simulink model "bolide_complet"  (R2023b)
settings: Solver=VariableStepAuto  StartTime=0.0  StopTime=50  RelTol=1e-3
model workspace (MATLAB code in the model file):
  | % Paramètres du système
  | mb = 0.7;
  | mw = 0.1;
  | Ix = 0.001;
  | Iz = 0.001;
  | Iwx = 0.001;
  | Iwy = 0.001;
  | Iwz = 0.001;
  | l = 0.22;
  | d = 0.2;
  | R = 2.05;
  | k = 0.258;
  | rho = 0.04;
  | 
  | % A l'équilibre
  | 
  | ubar = 1;
  | psibar = 0;
libraries: slpidlib x2

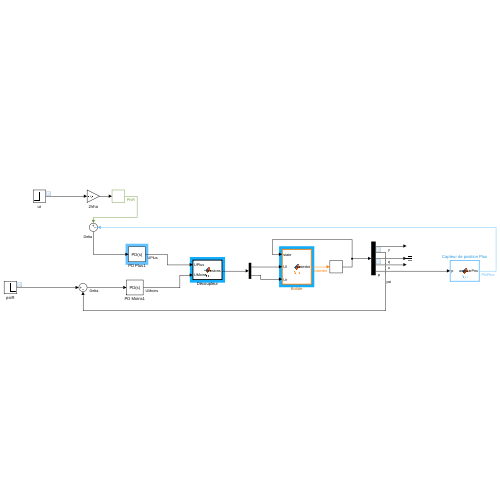
[thumbnail: Simulink's stored preview of the top-level diagram]
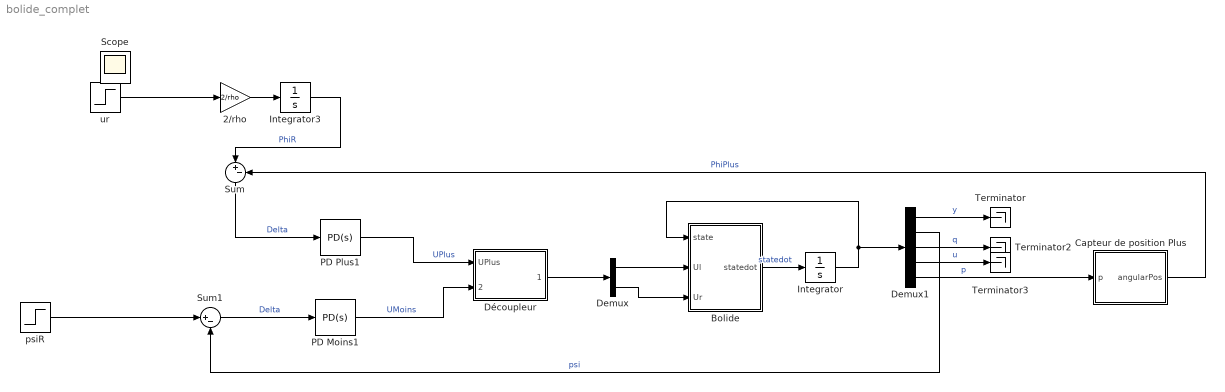
== system bolide_complet ==
  2/rho : Gain  Gain=2/rho
  Bolide : MATLAB Function  TreatAsAtomicUnit=on
  Capteur de position Plus : MATLAB Function  TreatAsAtomicUnit=on
  Demux : Demux  Outputs=2
  Demux1 : Demux  Outputs=5
  Découpleur : MATLAB Function  TreatAsAtomicUnit=on
  Integrator : Integrator
  Integrator3 : Integrator
  PD Moins1 : slpidlib/PID Controller  Controller=PD  Form=Parallel  TimeDomain=Continuous-time  UseExternalTs=off  SampleTime=-1  IntegratorMethod=Forward Euler  FilterMethod=Forward Euler  ControllerParametersSource=internal  P=12.6058302791515  I=497413215071.165  UseKiTs=off  D=1.80702520106984  N=1442.48241498748  UseFilter=on  TunerSelectOption=Transfer Function Based (PID Tuner App)  InitialConditionSource=internal  InitialConditionForIntegrator=0  InitialConditionForFilter=0  DifferentiatorICPrevScaledInput=0  ExternalReset=none  TrackingMode=off  Kt=1  LimitOutput=off  SatLimitsSource=internal  UpperSaturationLimit=inf  LowerSaturationLimit=-inf  LinearizeAsGain=on  AntiWindupMode=none  Kb=1  LimitIntegrator=off  UpperIntegratorSaturationLimit=inf  LowerIntegratorSaturationLimit=-inf  POutMin=[]  POutMax=[]  IOutMin=[]  IOutMax=[]  DOutMin=[]  DOutMax=[]  NOutMin=[]  NOutMax=[]  SumOutMin=[]  SumOutMax=[]  SaturationOutMin=[]  SaturationOutMax=[]  PParamMin=[]  PParamMax=[]  IParamMin=[]  IParamMax=[]  DParamMin=[]  DParamMax=[]  NParamMin=[]  NParamMax=[]  KbParamMin=[]  KbParamMax=[]  KtParamMin=[]  KtParamMax=[]  KbOutMin=[]  KbOutMax=[]  KtOutMin=[]  KtOutMax=[]  IntegratorOutMin=[]  IntegratorOutMax=[]  FilterOutMin=[]  FilterOutMax=[]  SumI1OutMin=[]  SumI1OutMax=[]  SumI2OutMin=[]  SumI2OutMax=[]  SumI3OutMin=[]  SumI3OutMax=[]  SumI4OutMin=[]  SumI4OutMax=[]  SumDOutMin=[]  SumDOutMax=[]  DifferentiatorOutMin=[]  DifferentiatorOutMax=[]  FilterDiffOutCoefMin=[]  FilterDiffOutCoefMax=[]  ReciprocalOutMin=[]  ReciprocalOutMax=[]  SumDenOutMin=[]  SumDenOutMax=[]  SumNumOutMin=[]  SumNumOutMax=[]  DivideOutMin=[]  DivideOutMax=[]  UdiffTsProdOutMin=[]  UdiffTsProdOutMax=[]  NTsProdOutMin=[]  NTsProdOutMax=[]  UintegralTsProdOutMin=[]  UintegralTsProdOutMax=[]  UngainTsProdOutMin=[]  UngainTsProdOutMax=[]  ClampingZeroOutDataTypeStr=Inherit: Inherit via back propagation  ClampingZeroOutMin=[]  ClampingZeroOutMax=[]  FilterDenConstantOutDataTypeStr=Inherit: Inherit via back propagation  FilterDenConstantOutMin=[]  FilterDenConstantOutMax=[]  PCopyOutDataTypeStr=Inherit: Inherit via back propagation  PCopyOutMin=[]  PCopyOutMax=[]  NCopyOutDataTypeStr=Inherit: Inherit via back propagation  NCopyOutMin=[]  NCopyOutMax=[]  IntegratorContinuousStateAttributes=''  IntegratorStateMustResolveToSignalObject=off  IntegratorRTWStateStorageClass=Auto  FilterContinuousStateAttributes=''  FilterStateMustResolveToSignalObject=off  FilterRTWStateStorageClass=Auto  ParallelPVariant=InternalParameters  IdealPVariant=Disabled  IVariant=Disabled  DVariant=InternalParameters  IntegratorVariant=Disabled  SatVariant=Disabled  AWVariant=Disabled  PCopyVariant=Disabled  TRVariant=Disabled  FdbkBlocksVariant=Forward  IdealPFdbkVariant=Disabled  SatFdbkVariant=Disabled  DerivativeFilterVariant=ContFilter  NVariant=InternalParameters  NCopyVariant=Disabled  FilterICVariant=InternalICsFilter  IntegratorICVariant=Disabled  ExternalResetVariant=Disabled  TRSumVariant=Passthrough  SumFdbkVariant=Disabled  SumVariant=Sum_PD  TsampFilterVariant=InternalTs  TsampNgainVariant=Passthrough  TsampIntegralVariant=Disabled_SignalSpec  ExternalSaturationOutDataTypeStr=Inherit: Same as second input
  PD Plus1 : slpidlib/PID Controller  Controller=PD  Form=Parallel  TimeDomain=Continuous-time  UseExternalTs=off  SampleTime=-1  IntegratorMethod=Forward Euler  FilterMethod=Forward Euler  ControllerParametersSource=internal  P=2.31142819167864  I=1  UseKiTs=off  D=0.156652355088966  N=38.0509122005018  UseFilter=on  TunerSelectOption=Transfer Function Based (PID Tuner App)  InitialConditionSource=internal  InitialConditionForIntegrator=0  InitialConditionForFilter=0  DifferentiatorICPrevScaledInput=0  ExternalReset=none  TrackingMode=off  Kt=1  LimitOutput=off  SatLimitsSource=internal  UpperSaturationLimit=inf  LowerSaturationLimit=-inf  LinearizeAsGain=on  AntiWindupMode=none  Kb=1  LimitIntegrator=off  UpperIntegratorSaturationLimit=inf  LowerIntegratorSaturationLimit=-inf  POutMin=[]  POutMax=[]  IOutMin=[]  IOutMax=[]  DOutMin=[]  DOutMax=[]  NOutMin=[]  NOutMax=[]  SumOutMin=[]  SumOutMax=[]  SaturationOutMin=[]  SaturationOutMax=[]  PParamMin=[]  PParamMax=[]  IParamMin=[]  IParamMax=[]  DParamMin=[]  DParamMax=[]  NParamMin=[]  NParamMax=[]  KbParamMin=[]  KbParamMax=[]  KtParamMin=[]  KtParamMax=[]  KbOutMin=[]  KbOutMax=[]  KtOutMin=[]  KtOutMax=[]  IntegratorOutMin=[]  IntegratorOutMax=[]  FilterOutMin=[]  FilterOutMax=[]  SumI1OutMin=[]  SumI1OutMax=[]  SumI2OutMin=[]  SumI2OutMax=[]  SumI3OutMin=[]  SumI3OutMax=[]  SumI4OutMin=[]  SumI4OutMax=[]  SumDOutMin=[]  SumDOutMax=[]  DifferentiatorOutMin=[]  DifferentiatorOutMax=[]  FilterDiffOutCoefMin=[]  FilterDiffOutCoefMax=[]  ReciprocalOutMin=[]  ReciprocalOutMax=[]  SumDenOutMin=[]  SumDenOutMax=[]  SumNumOutMin=[]  SumNumOutMax=[]  DivideOutMin=[]  DivideOutMax=[]  UdiffTsProdOutMin=[]  UdiffTsProdOutMax=[]  NTsProdOutMin=[]  NTsProdOutMax=[]  UintegralTsProdOutMin=[]  UintegralTsProdOutMax=[]  UngainTsProdOutMin=[]  UngainTsProdOutMax=[]  ClampingZeroOutDataTypeStr=Inherit: Inherit via back propagation  ClampingZeroOutMin=[]  ClampingZeroOutMax=[]  FilterDenConstantOutDataTypeStr=Inherit: Inherit via back propagation  FilterDenConstantOutMin=[]  FilterDenConstantOutMax=[]  PCopyOutDataTypeStr=Inherit: Inherit via back propagation  PCopyOutMin=[]  PCopyOutMax=[]  NCopyOutDataTypeStr=Inherit: Inherit via back propagation  NCopyOutMin=[]  NCopyOutMax=[]  IntegratorContinuousStateAttributes=''  IntegratorStateMustResolveToSignalObject=off  IntegratorRTWStateStorageClass=Auto  FilterContinuousStateAttributes=''  FilterStateMustResolveToSignalObject=off  FilterRTWStateStorageClass=Auto  ParallelPVariant=InternalParameters  IdealPVariant=Disabled  IVariant=Disabled  DVariant=InternalParameters  IntegratorVariant=Disabled  SatVariant=Disabled  AWVariant=Disabled  PCopyVariant=Disabled  TRVariant=Disabled  FdbkBlocksVariant=Forward  IdealPFdbkVariant=Disabled  SatFdbkVariant=Disabled  DerivativeFilterVariant=ContFilter  NVariant=InternalParameters  NCopyVariant=Disabled  FilterICVariant=InternalICsFilter  IntegratorICVariant=Disabled  ExternalResetVariant=Disabled  TRSumVariant=Passthrough  SumFdbkVariant=Disabled  SumVariant=Sum_PD  TsampFilterVariant=InternalTs  TsampNgainVariant=Passthrough  TsampIntegralVariant=Disabled_SignalSpec  ExternalSaturationOutDataTypeStr=Inherit: Same as second input
  Sum : Sum  Inputs=|+-
  Sum1 : Sum  Inputs=|+-
  Terminator : Terminator
  Terminator2 : Terminator
  Terminator3 : Terminator
  psiR : Step  Time=10  Before=10  After=psibar  SampleTime=0
  ur : Step  Time=5  After=ubar  SampleTime=0
  Scope : Scope
  wires:
  Découpleur/1(tensions) -> Demux/1
  Demux/1 -> Bolide/2(Ul)
  Demux/2 -> Bolide/3(Ur)
  PD Plus1/1 -> Découpleur/1(UPlus)  "UPlus"
  Bolide/1(statedot) -> Integrator/1  "statedot"
  Integrator/1 -> Bolide/1(state), Demux1/1
  Demux1/1 -> Terminator/1  "y"
  Demux1/2 -> Sum1/2  "psi"
  Demux1/3 -> Terminator2/1  "q"
  Demux1/4 -> Terminator3/1  "u"
  Demux1/5 -> Capteur de position Plus/1(p)  "p"
  Sum/1 -> PD Plus1/1  "Delta"
  Capteur de position Plus/1(angularPos) -> Sum/2  "PhiPlus"
  2/rho/1 -> Integrator3/1
  Integrator3/1 -> Sum/1  "PhiR"
  Sum1/1 -> PD Moins1/1  "Delta"
  psiR/1 -> Sum1/1
  ur/1 -> 2/rho/1
  PD Moins1/1 -> Découpleur/2(UMoins)  "UMoins"

== matlab function bolide_complet/Découpleur ==
  data: UPlus input; tensions output; UMoins input
function tensions = fcn(UPlus, UMoins)

Ur = (UPlus + UMoins)/2;
Ul = (UPlus - UMoins)/2;

tensions = [Ul; Ur];

== matlab function bolide_complet/Bolide ==
  data: state input size=[5 1]; statedot output; Ul input; Ur input; mb parameter; mw parameter; Ix parameter; Iz parameter; Iwx parameter; Iwy parameter; Iwz parameter; l parameter; d parameter; R parameter; k parameter; rho parameter
function statedot = fcn(state, Ul, Ur, mb, mw, Ix, Iz, Iwx, Iwy, Iwz, l, d, R, k, rho)

% Variables d'état
y = state(1);
psi = state(2);
q = state(3);
u = state(4);
p = state(5);

% Ecritures simplifiées
M = mb + 2*mw;
Ipsi = Ix + Iwx + Iz + Iwz + mw*((l*l)/2) + Iwy*(l*l)/(2*rho*rho);
alpha = M + 2*Iwy/(rho*rho);
beta = Ipsi + mb*d*d;
mu1 = (l*k)/(2*beta*rho*R);
mu2 = (mb*d)/beta;
mu3 = k/(alpha*rho*R);
mu4 = (mb*d)/alpha;


% Equations de fonctionnement
ydot = u*sin(psi);
psidot = q;
qdot = mu1*(Ur-Ul-(k*l*q)/rho) + mu2*u*q;
udot = mu3*(Ur+Ul-(2*k*u)/rho) - mu4*q*q;
pdot = u;

statedot = [ydot; psidot; qdot; udot; pdot];

== matlab function bolide_complet/Capteur de position Plus ==
  data: p input; angularPos output; rho parameter
function angularPos = fcn(p,rho)

phiPlus = (2*p)/rho;

angularPos = phiPlus;
